simulink model "gui1"  (R2015a)
settings: Solver=ode45  StartTime=0.0  StopTime=30  RelTol=1e-3
values from neighbouring files (symbols this model uses):
  control_value = str2double(get(hObject,'String'))    [gui2.m]    (also in parameters.m = deg2rad(15))
  tau_max = 5    [parameters.m]
undefined symbols (not defined in the file or in its folder): setpoint
libraries: dspquant2 x2, dspstat3 x1
settings Model: Creator=preston  LastModifiedBy=Nathan

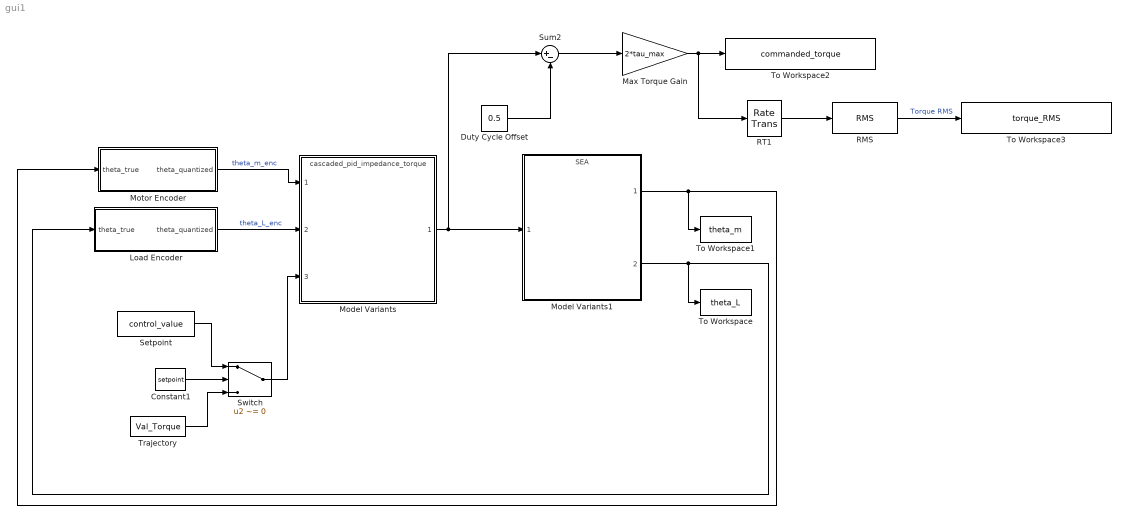
== system gui1 ==
  Constant1 : Constant  Value=setpoint
  Duty Cycle Offset : Constant  Value=0.5
  Load Encoder : Subsystem
  Max Torque Gain : Gain  Gain=2*tau_max
  Model Variants : ModelReference  ModelNameDialog=cascaded_pid_impedance_torque.slx  Variant=on  ModelReferenceVersion=1.39  CopyOfModelName=cascaded_pid_impedance_torque.slx  DefaultDataLogging=on
      settings: AttributesFormatString=%<ActiveVariant>
  Model Variants1 : ModelReference  ModelNameDialog=SEA.slx  SimulationMode=Normal  Variant=on  ModelReferenceVersion=1.12  CopyOfModelName=SEA.slx  DefaultDataLogging=on
      settings: AttributesFormatString=%<ActiveVariant>
  Motor Encoder : Subsystem
  RMS : dspstat3/RMS  run=on  reset_popup=None  InputProcessing=Columns as channels (frame based)  directionMode=Each column  dimension=1  treatSBRowAsCol=off
  RT1 : RateTransition  OutPortSampleTime=T_sample_control
  Setpoint : Constant  Value=control_value
  Sum2 : Sum  Inputs=|+-
  Switch : Switch  Criteria=u2 ~= 0
  To Workspace : ToWorkspace  VariableName=theta_L  SaveFormat=Structure With Time  SampleTime=-1
  To Workspace1 : ToWorkspace  VariableName=theta_m  SaveFormat=Structure With Time  SampleTime=-1
  To Workspace2 : ToWorkspace  VariableName=commanded_torque  SaveFormat=Structure With Time  SampleTime=-1
  To Workspace3 : ToWorkspace  VariableName=torque_RMS  SaveFormat=Structure With Time  SampleTime=-1
  Trajectory : FromWorkspace  VariableName=Val_Torque  OutputAfterFinalValue=Holding final value
  wires:
  Model Variants1/1 -> Motor Encoder/1(theta_true), To Workspace1/1
  Model Variants1/2 -> Load Encoder/1(theta_true), To Workspace/1
  Model Variants/1 -> Sum2/1, Model Variants1/1
  Duty Cycle Offset/1 -> Sum2/2
  Sum2/1 -> Max Torque Gain/1
  Max Torque Gain/1 -> RT1/1, To Workspace2/1
  RMS/1 -> To Workspace3/1  "Torque RMS"
  Switch/1 -> Model Variants/3
  Setpoint/1 -> Switch/1
  Trajectory/1 -> Switch/3
  Constant1/1 -> Switch/2
  RT1/1 -> RMS/1
  Motor Encoder/1(theta_quantized) -> Model Variants/1  "theta_m_enc"
  Load Encoder/1(theta_quantized) -> Model Variants/2  "theta_L_enc"

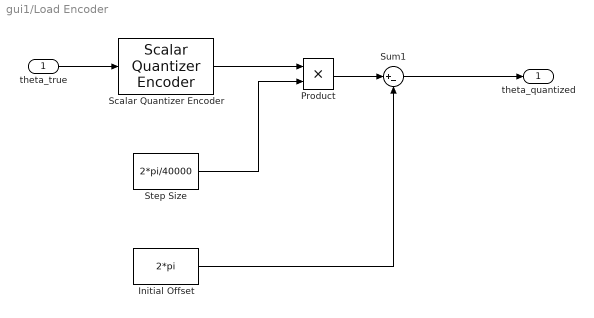
== system gui1/Load Encoder ==
  theta_true : Inport
  Initial Offset : Constant  Value=2*pi
  Product : Product
  Scalar Quantizer Encoder : dspquant2/Scalar Quantizer Encoder  paramSrc=Specify via dialog  partType=Bounded  BBoundary=[-2*pi:2*pi/40000:2*pi]  UBoundary=[2:9]  SearchMethod=Binary  tieBreakRule=Choose the lower index  outQU=off  outQError=off  codebook=[-2*pi+pi/10000:2*pi/10000:2*pi]  outStatus=off  invalidin=Clip and warn  idtype=int32  roundingMode=Floor  overflowMode=off
  Step Size : Constant  Value=2*pi/40000
  Sum1 : Sum  Inputs=|+-
  theta_quantized : Outport
  wires:
  theta_true/1 -> Scalar Quantizer Encoder/1
  Scalar Quantizer Encoder/1 -> Product/1
  Step Size/1 -> Product/2
  Product/1 -> Sum1/1
  Initial Offset/1 -> Sum1/2
  Sum1/1 -> theta_quantized/1

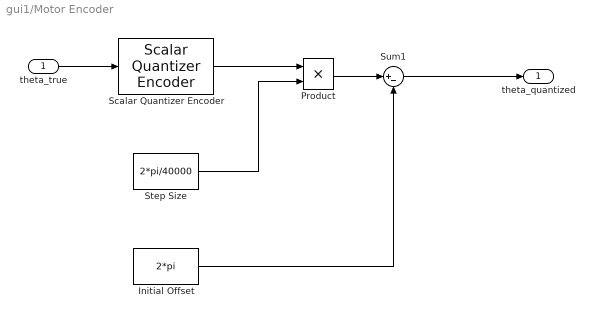
== system gui1/Motor Encoder ==
  theta_true : Inport
  Initial Offset : Constant  Value=2*pi
  Product : Product
  Scalar Quantizer Encoder : dspquant2/Scalar Quantizer Encoder  paramSrc=Specify via dialog  partType=Bounded  BBoundary=[-2*pi:2*pi/40000:2*pi]  UBoundary=[2:9]  SearchMethod=Binary  tieBreakRule=Choose the lower index  outQU=off  outQError=off  codebook=[-2*pi+pi/10000:2*pi/10000:2*pi]  outStatus=off  invalidin=Clip and warn  idtype=int32  roundingMode=Floor  overflowMode=off
  Step Size : Constant  Value=2*pi/40000
  Sum1 : Sum  Inputs=|+-
  theta_quantized : Outport
  wires:
  theta_true/1 -> Scalar Quantizer Encoder/1
  Scalar Quantizer Encoder/1 -> Product/1
  Step Size/1 -> Product/2
  Product/1 -> Sum1/1
  Initial Offset/1 -> Sum1/2
  Sum1/1 -> theta_quantized/1
